simulink model "Test_Cart_Path_Logic_Flow_2021"  (R2021a)
settings: Solver=VariableStepAuto  StartTime=0.0  StopTime=stopTime  RelTol=1e-3
PreLoadFcn:
  | initializeParameters
InitFcn:
  | initializeParameters
StartFcn:
  | initializeParameters
undefined symbols (not defined in the file): bale, baleParam, cart, cartParam, contactGripper, floorParam, manip, TsCtrl, X, Y, Z
libraries: sm_lib x216, nesl_utility x30, fl_lib x4, robotcorelib x2, robotmaniplib x2, simulink x2, Multibody_Multiphysics_Lib x2
(part 1 of 6)
settings Model: Creator=sabir  LastModifiedBy=sabir
settings DebuggingCC: UnconnectedInputMsg=none  UnconnectedOutputMsg=none  UnconnectedLineMsg=none
settings ModelReferenceCC: EnableRefExpFcnMdlSchedulingChecks=off
settings RTWCC: Description=Generic Real-Time Target  DLArmComputeVersion=20.02.1

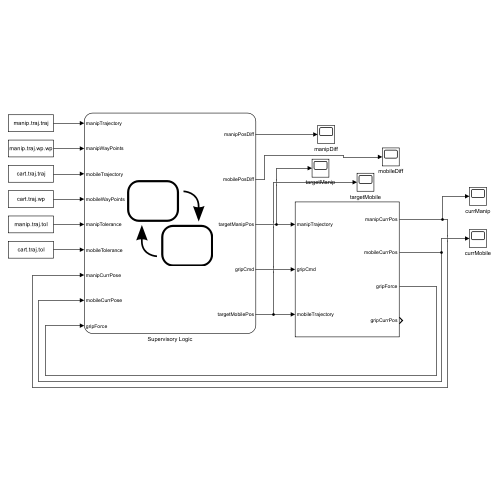
[thumbnail: Simulink's stored preview of the top-level diagram]
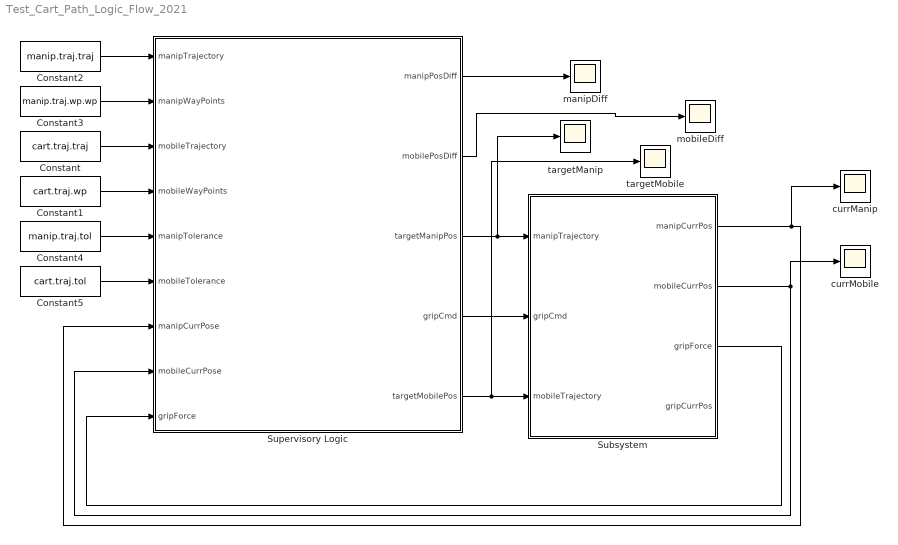
== system Test_Cart_Path_Logic_Flow_2021 ==
  Constant : Constant  Value=cart.traj.traj
  Constant1 : Constant  Value=cart.traj.wp
  Constant2 : Constant  Value=manip.traj.traj
  Constant3 : Constant  Value=manip.traj.wp.wp
  Constant4 : Constant  Value=manip.traj.tol
  Constant5 : Constant  Value=cart.traj.tol
  Subsystem : Subsystem
  Supervisory Logic : Stateflow chart  TreatAsAtomicUnit=on
      settings: PortSchema="{\"entries\":[{\"content\":{\"sides\":[{\"content\":{\"connectorIds\":[\"In2\",\"In7\",\"In4\",\"In6\",\"In8\",\"In9\",\"In3\",\"In5\",\"In1\"]},\"type\":\"ConnectorPlacement.EquallySpacedRectSide\",\"uuid\":\"1b49e4dc-4524-494e-96ea-732cb30677b8\"},{\"content\":{\"connectorIds\":[\"Out3\",\"Out4\",\"Out2\",\"Out1\",\"Out5\"],\"side\":\"RIGHT\"},\"type\":\"ConnectorPlacement.EquallySpacedRectSide\",\"uuid\":\"5c4135dd-083d-443e-ad50-3d8d6c2ff107\"},{\"content\":{\"side\":\"TOP\"},\"type\":\"ConnectorPlacement.EquallySpacedRectSide\",\"uuid\":\"6984522e-9a4c-46f1-a304-2147c16b45bd\"}]},\"type\":\"ConnectorPlacement.EquallySpacedConnector\",\"uuid\":\"7c7877d4-26a8-4ce7-8b0a-2214cf03121b\"}],\"packageUris\":[\"http://schema.mathworks.com/mf0/Connector/R2020b\"],\"version\":\"1.0\"}"
  currManip : Scope
  currMobile : Scope
  manipDiff : Scope
  mobileDiff : Scope
  targetManip : Scope
  targetMobile : Scope
  wires:
  Supervisory Logic/2(targetManipPos) -> targetManip/1, Subsystem/1(manipTrajectory)
  Supervisory Logic/5(targetMobilePos) -> targetMobile/1, Subsystem/3(mobileTrajectory)
  Supervisory Logic/1(gripCmd) -> Subsystem/2(gripCmd)
  Subsystem/1(manipCurrPos) -> currManip/1, Supervisory Logic/3(manipCurrPose)
  Subsystem/2(mobileCurrPos) -> Supervisory Logic/5(mobileCurrPose), currMobile/1
  Subsystem/3(gripForce) -> Supervisory Logic/1(gripForce)
  Constant1/1 -> Supervisory Logic/6(mobileWayPoints)
  Constant4/1 -> Supervisory Logic/8(manipTolerance)
  Constant5/1 -> Supervisory Logic/9(mobileTolerance)
  Constant/1 -> Supervisory Logic/4(mobileTrajectory)
  Constant3/1 -> Supervisory Logic/7(manipWayPoints)
  Constant2/1 -> Supervisory Logic/2(manipTrajectory)
  Supervisory Logic/3(manipPosDiff) -> manipDiff/1
  Supervisory Logic/4(mobilePosDiff) -> mobileDiff/1

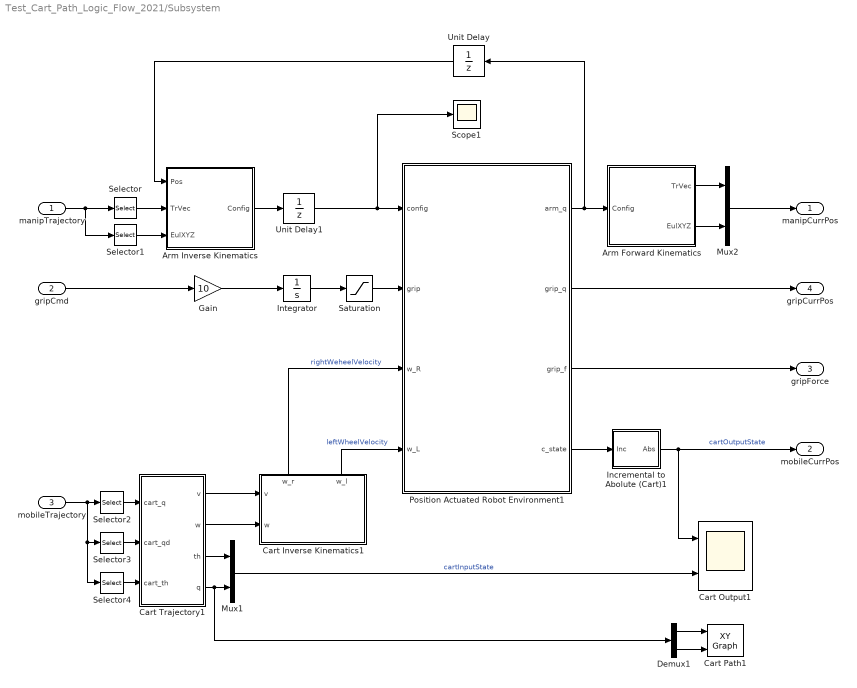
== system Test_Cart_Path_Logic_Flow_2021/Subsystem ==
  manipTrajectory : Inport
  gripCmd : Inport  Port=2
  mobileTrajectory : Inport  Port=3
  Arm Forward Kinematics : Subsystem
  Arm Inverse Kinematics : Subsystem
  Cart Inverse Kinematics1 : Subsystem
      settings: PortSchema="{\"entries\":[{\"content\":{\"sides\":[{\"content\":{\"connectorIds\":[\"In1\",\"In2\"]},\"type\":\"ConnectorPlacement.EquallySpacedRectSide\",\"uuid\":\"7f22b938-58ee-4238-b1b7-b23dabfa1fc4\"},{\"content\":{\"side\":\"RIGHT\"},\"type\":\"ConnectorPlacement.EquallySpacedRectSide\",\"uuid\":\"1a095504-1358-40ea-b561-93851aaa8a0a\"},{\"content\":{\"connectorIds\":[\"Out1\",\"Out2\"],\"side\":\"TOP\"},\"type\":\"ConnectorPlacement.EquallySpacedRectSide\",\"uuid\":\"86fe0244-d864-449d-a01f-840e24c5bd93\"}]},\"type\":\"ConnectorPlacement.EquallySpacedConnector\",\"uuid\":\"92036445-0dba-4b1c-875d-58a31873dca2\"}],\"packageUris\":[\"http://schema.mathworks.com/mf0/Connector/R2020b\"],\"version\":\"1.0\"}"
  Cart Output1 : Scope  NumInputPorts=2
  Cart Path1 : simulink/Sinks/XY Graph  xmin=-1  xmax=1  ymin=-1  ymax=1  st=-1
  Cart Trajectory1 : Subsystem
  Demux1 : Demux  Outputs=2
  Gain : Gain  Gain=10
  Incremental to Abolute (Cart)1 : Subsystem
  Integrator : Integrator
  Mux1 : Mux  Inputs=2
  Mux2 : Mux  Inputs=2
  Position Actuated Robot Environment1 : Subsystem  AutoFrameSizeCalculation=on
  Saturation : Saturate  UpperLimit=0.07  LowerLimit=0
  Scope1 : Scope
  Selector : Selector  InputPortWidth=6  IndexOptions=Index vector (dialog)  Indices=[1:3]  OutputSizes=1
  Selector1 : Selector  InputPortWidth=6  IndexOptions=Index vector (dialog)  Indices=[4:6]  OutputSizes=1
  Selector2 : Selector  InputPortWidth=4  IndexOptions=Index vector (dialog)  Indices=[1:2]  OutputSizes=1
  Selector3 : Selector  InputPortWidth=4  IndexOptions=Index vector (dialog)  Indices=3  OutputSizes=1
  Selector4 : Selector  InputPortWidth=4  IndexOptions=Index vector (dialog)  Indices=4  OutputSizes=1
  Unit Delay : UnitDelay  SampleTime=-1  HasFrameUpgradeWarning=on
  Unit Delay1 : UnitDelay  SampleTime=TsCtrl/5  HasFrameUpgradeWarning=on
  manipCurrPos : Outport
  mobileCurrPos : Outport  Port=2
  gripForce : Outport  Port=3
  gripCurrPos : Outport  Port=4
  wires:
  Mux1/1 -> Cart Output1/2  "cartInputState"
  Unit Delay/1 -> Arm Inverse Kinematics/1(Pos)
  manipTrajectory/1 -> Selector1/1, Selector/1
  Cart Inverse Kinematics1/1(w_r) -> Position Actuated Robot Environment1/3(w_R)  "rightWeheelVelocity"
  Selector3/1 -> Cart Trajectory1/2(cart_qd)
  mobileTrajectory/1 -> Selector2/1, Selector4/1, Selector3/1
  Integrator/1 -> Saturation/1
  Demux1/1 -> Cart Path1/1
  Position Actuated Robot Environment1/2(grip_q) -> gripCurrPos/1
  gripCmd/1 -> Gain/1
  Selector2/1 -> Cart Trajectory1/1(cart_q)
  Selector4/1 -> Cart Trajectory1/3(cart_th)
  Arm Inverse Kinematics/1(Config) -> Unit Delay1/1
  Incremental to Abolute (Cart)1/1(Abs) -> mobileCurrPos/1, Cart Output1/1  "cartOutputState"
  Arm Forward Kinematics/1(TrVec) -> Mux2/1
  Saturation/1 -> Position Actuated Robot Environment1/2(grip)
  Cart Trajectory1/4(q) -> Demux1/1, Mux1/2
  Position Actuated Robot Environment1/1(arm_q) -> Arm Forward Kinematics/1(Config), Unit Delay/1
  Demux1/2 -> Cart Path1/2
  Cart Trajectory1/1(v) -> Cart Inverse Kinematics1/1(v)
  Position Actuated Robot Environment1/3(grip_f) -> gripForce/1
  Arm Forward Kinematics/2(EulXYZ) -> Mux2/2
  Mux2/1 -> manipCurrPos/1
  Selector1/1 -> Arm Inverse Kinematics/3(EulXYZ)
  Cart Trajectory1/2(w) -> Cart Inverse Kinematics1/2(w)
  Position Actuated Robot Environment1/4(c_state) -> Incremental to Abolute (Cart)1/1(Inc)
  Cart Inverse Kinematics1/2(w_l) -> Position Actuated Robot Environment1/4(w_L)  "leftWheelVelocity"
  Cart Trajectory1/3(th) -> Mux1/1
  Selector/1 -> Arm Inverse Kinematics/2(TrVec)
  Unit Delay1/1 -> Position Actuated Robot Environment1/1(config), Scope1/1
  Gain/1 -> Integrator/1

== system Test_Cart_Path_Logic_Flow_2021/Subsystem/Arm Forward Kinematics ==
  Config : Inport
  Coordinate Transformation Conversion : robotcorelib/Coordinate Transformation Conversion  InputRepresentation=Homogeneous Transformation  InputEulerSequence=ZYX  ShowTrVecInputPort=on  OutputRepresentation=Euler Angles  OutputEulerSequence=XYZ  ShowTrVecOutputPort=on  SimulateUsing=Interpreted execution
  Gain : Gain  Gain=-1
  Get Transform : robotmaniplib/Get Transform  RigidBodyTree=manipulator_tree  SourceBody=Base  TargetBody=Body7  SimulateUsing=Interpreted execution
  TrVec : Outport
  EulXYZ : Outport  Port=2
  wires:
  Get Transform/1 -> Coordinate Transformation Conversion/1
  Config/1 -> Get Transform/1
  Coordinate Transformation Conversion/2 -> Gain/1
  Gain/1 -> TrVec/1
  Coordinate Transformation Conversion/1 -> EulXYZ/1

== system Test_Cart_Path_Logic_Flow_2021/Subsystem/Arm Inverse Kinematics ==
  Pos : Inport
  TrVec : Inport  Port=2
  EulXYZ : Inport  Port=3
  Constant2 : Constant  Value=[1 1 1 1 1 1]
  Coordinate Transformation Conversion : robotcorelib/Coordinate Transformation Conversion  InputRepresentation=Euler Angles  InputEulerSequence=XYZ  ShowTrVecInputPort=on  OutputRepresentation=Homogeneous Transformation  OutputEulerSequence=ZYX  ShowTrVecOutputPort=on  SimulateUsing=Code generation
  Inverse Kinematics : robotmaniplib/Inverse Kinematics  RigidBodyTree=manipulator_tree  EndEffector=Body7  ShowInfo=on  SolverName=BFGS Gradient Projection  EnforceJointLimits=on  MaxIterations=50  MaxTime=3  GradientTolerance=1e-7  SolutionTolerance=1e-6  StepTolerance=1e-12  ErrorChangeTolerance=1e-6  UseErrorDamping=on  DampingBias=0.0025  SimulateUsing=Code generation
  Transpose : Math  Operator=transpose  SaturateOnIntegerOverflow=on
  Config : Outport
  wires:
  Inverse Kinematics/1 -> Config/1
  Constant2/1 -> Inverse Kinematics/2
  Transpose/1 -> Inverse Kinematics/3
  EulXYZ/1 -> Coordinate Transformation Conversion/1
  TrVec/1 -> Coordinate Transformation Conversion/2
  Coordinate Transformation Conversion/1 -> Inverse Kinematics/1
  Pos/1 -> Transpose/1

== system Test_Cart_Path_Logic_Flow_2021/Subsystem/Cart Inverse Kinematics1 ==
  v : Inport
  w : Inport  Port=2
  Mux : Mux  Inputs=2
  cartTraj2Signal : Subsystem
  w_r : Outport
  w_l : Outport  Port=2
  wires:
  w/1 -> Mux/2
  v/1 -> Mux/1
  Mux/1 -> cartTraj2Signal/1(u)
  cartTraj2Signal/1(w_r) -> w_r/1
  cartTraj2Signal/2(w_l) -> w_l/1

== system Test_Cart_Path_Logic_Flow_2021/Subsystem/Cart Trajectory1 ==
  cart_q : Inport
  cart_qd : Inport  Port=2
  cart_th : Inport  Port=3
  Discrete Derivative : simulink/Discrete/Discrete Derivative  gainval=1.0  ICPrevScaledInput=0.0  OutMin=[]  OutMax=[]  OutDataType=fixdt(1, 16)  OutScaling=2^-10  DoSatur=off
  Gain : Gain  Gain=-1
  v : Outport
  w : Outport  Port=2
  th : Outport  Port=3
  q : Outport  Port=4
  wires:
  cart_th/1 -> th/1, Discrete Derivative/1
  cart_q/1 -> q/1
  cart_qd/1 -> v/1
  Discrete Derivative/1 -> Gain/1
  Gain/1 -> w/1

== system Test_Cart_Path_Logic_Flow_2021/Subsystem/Incremental to Abolute (Cart)1 ==
  Inc : Inport
  Constant : Constant  Value=[cartParam.Initial.X cartParam.Initial.Y cartParam.Initial.Phase]
  Sum : Sum  Inputs=|++
  Abs : Outport
  wires:
  Constant/1 -> Sum/2
  Inc/1 -> Sum/1
  Sum/1 -> Abs/1

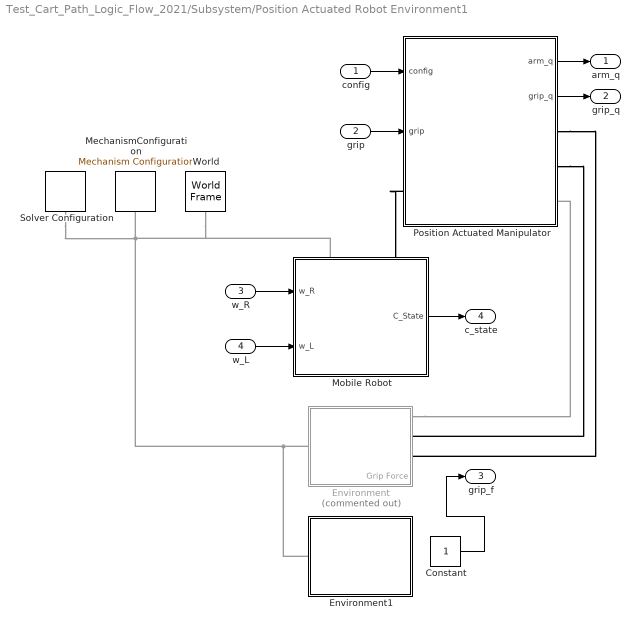
== system Test_Cart_Path_Logic_Flow_2021/Subsystem/Position Actuated Robot Environment1 ==
  config : Inport
  grip : Inport  Port=2
  w_R : Inport  Port=3
  w_L : Inport  Port=4
  Constant : Constant
  Environment : Subsystem  Commented=on  AutoFrameSizeCalculation=on
      settings: PortSchema="{\"entries\":[{\"content\":{\"sides\":[{\"content\":{\"connectorIds\":[\"LConn1\"]},\"type\":\"ConnectorPlacement.EquallySpacedRectSide\",\"uuid\":\"231e75f1-a9d1-4ad8-a62d-f4afe3591ae3\"},{\"content\":{\"connectorIds\":[\"RConn1\",\"RConn2\",\"RConn3\",\"Out1\"],\"side\":\"RIGHT\"},\"type\":\"ConnectorPlacement.EquallySpacedRectSide\",\"uuid\":\"58308121-f635-4820-a5b0-daa09c396c96\"},{\"content\":{\"side\":\"TOP\"},\"type\":\"ConnectorPlacement.EquallySpacedRectSide\",\"uuid\":\"269f5f23-d385-4e8d-96a8-2b8b856304b4\"}]},\"type\":\"ConnectorPlacement.EquallySpacedConnector\",\"uuid\":\"239c6083-2cec-4eff-aa6f-62c0a8160f9f\"}],\"packageUris\":[\"http://schema.mathworks.com/mf0/Connector/R2020b\"],\"version\":\"1.0\"}"
  Environment1 : Subsystem
  MechanismConfiguration : sm_lib/Utilities/Mechanism Configuration  UniformGravity=Constant  GravityVector=[0 0 -9.80665]  GravityVectorUnits=m/s^2  LinearizationDelta=0.001  JointModeTransitionNonlinearIterations=2
  Mobile Robot : Subsystem
      settings: PortSchema="{\"entries\":[{\"content\":{\"sides\":[{\"content\":{\"connectorIds\":[\"In1\",\"In2\"]},\"type\":\"ConnectorPlacement.EquallySpacedRectSide\",\"uuid\":\"d865e24f-6e94-4741-8663-2233d7cc6fe3\"},{\"content\":{\"connectorIds\":[\"Out1\"],\"side\":\"RIGHT\"},\"type\":\"ConnectorPlacement.EquallySpacedRectSide\",\"uuid\":\"e7ebc92e-d028-4010-9d41-bb6c59c0597a\"},{\"content\":{\"connectorIds\":[\"LConn1\",\"LConn2\"],\"side\":\"TOP\"},\"type\":\"ConnectorPlacement.EquallySpacedRectSide\",\"uuid\":\"98a320eb-86e9-479f-99cc-19c49b219ef0\"}]},\"type\":\"ConnectorPlacement.EquallySpacedConnector\",\"uuid\":\"33108f5f-f594-4d41-bc94-cf092a0c20d2\"}],\"packageUris\":[\"http://schema.mathworks.com/mf0/Connector/R2020b\"],\"version\":\"1.0\"}"
  Position Actuated Manipulator : Subsystem
  Solver Configuration : nesl_utility/Solver Configuration  PhysicalDomain=network_engine_domain  SubClassName=solver  LeftPortType=input  RightPortType=generic  Tones=[]  Harmonics=[]  SimulateNoise=off  Profile=off  UseLocalSampling=off  EnableSwitchedLinearOptims=on  FrequencyDomain=off  UseCCode=off  RelTol=0.001  AbsTol=0.001  MinStep=1e-09  ToWorkspace=off  RevertToSquareIcSolve=off  NumHomotopyIterations=100  PhasorMode=off  PhasorModeNumHarmonics=1  ConsistencySolver=NEWTON_XTOL_AFTER_FTOL  IndexReductionMethod=DerivativeReplacement  DoDC=off  ResidualTolerance=1e-09  ConsistencyTolSource=GLOBAL  ConsistencyAbsTol=0.001  ConsistencyRelTol=0.001  ConsistencyTolFactor=0.001  UseLocalSolver=off  LocalSolverChoice=NE_BACKWARD_EULER_ADVANCER  ResolveIndetEquations=on  FunctionEvalNumThread=1  LocalSolverSampleTime=0.001  DoFixedCost=off  MaxNonlinIter=3  MaxModeIter=2  ComputeImpulses=off  ImpulseIterations=2  LinearAlgebra=Sparse  LinearAlgebraNumThread=0  EquationFormulation=NE_TIME_EF  DelaysMemoryBudget=10240  AutomaticFiltering=on  FilteringTimeConstant=filterCoeff  PartitionStorageMethod=AS_NEEDED  PartitionMemoryBudget=1024  PartitionMethod=ROBUST
  World : sm_lib/Frames and Transforms/World Frame
  arm_q : Outport
  grip_q : Outport  Port=2
  grip_f : Outport  Port=3
  c_state : Outport  Port=4
  wires:
  config/1 -> Position Actuated Manipulator/1(config)
  Position Actuated Manipulator/2(grip_q) -> grip_q/1
  Mobile Robot/1(C_State) -> c_state/1
  w_R/1 -> Mobile Robot/1(w_R)
  grip/1 -> Position Actuated Manipulator/2(grip)
  w_L/1 -> Mobile Robot/2(w_L)
  Position Actuated Manipulator/1(arm_q) -> arm_q/1
  Constant/1 -> grip_f/1
  connections:
  Environment/LConn1 -- Environment1/LConn1 -- Solver Configuration/RConn1 -- World/RConn1 -- Mobile Robot/LConn1 -- MechanismConfiguration/RConn1
  Position Actuated Manipulator/RConn2 -- Environment/RConn2
  Position Actuated Manipulator/RConn1 -- Environment/RConn3
  Position Actuated Manipulator/LConn1 -- Mobile Robot/LConn2
  Environment/RConn1 -- Position Actuated Manipulator/RConn3

== system Test_Cart_Path_Logic_Flow_2021/Subsystem/Cart Inverse Kinematics1/cartTraj2Signal ==
  u : Inport
  Constant : Constant  Value=cartParam.TireRadius
  Constant1 : Constant  Value=cartParam.DistanceBwTires
  cartTraj2Signal : MATLAB Function  TreatAsAtomicUnit=on
  w_r : Outport
  w_l : Outport  Port=2
  wires:
  cartTraj2Signal/2(w_l) -> w_l/1
  Constant/1 -> cartTraj2Signal/2(r)
  Constant1/1 -> cartTraj2Signal/3(b)
  u/1 -> cartTraj2Signal/1(u)
  cartTraj2Signal/1(w_r) -> w_r/1
